simulink model "lab1v3OrozcoBenavides"  (R2017b)
settings: Solver=VariableStepAuto  StartTime=0.0  StopTime=0.01  RelTol=1e-3
undefined symbols (not defined in the file or in its folder): DiscIntNeverNeededParam, magnitude
libraries: commchan3 x8, simulink_extras x7, commrandsrc3 x4, dsparch4 x2, simulink x1, commutil2 x1
settings Model: Creator=n0b0dy  LastModifiedBy=user

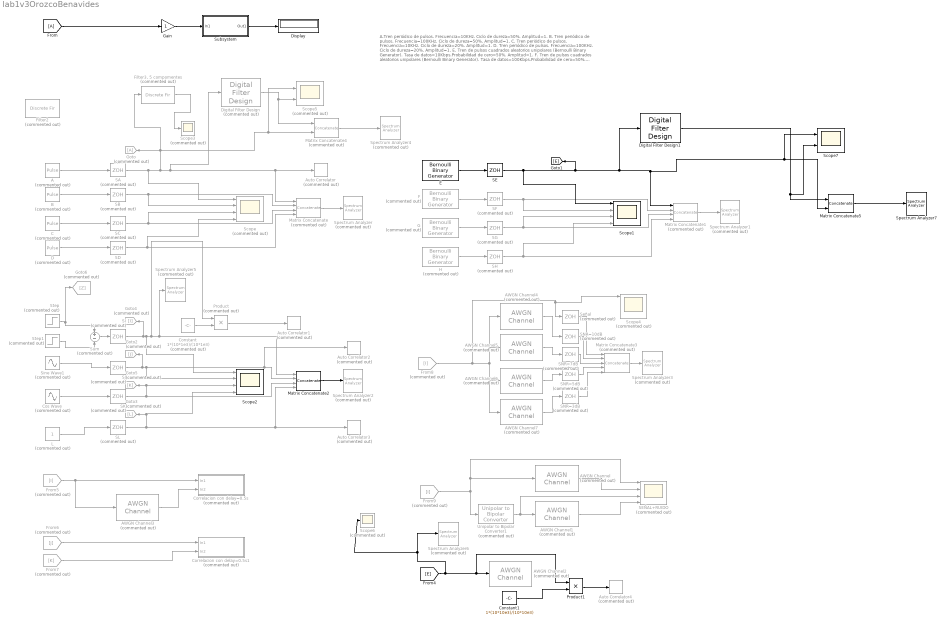
== system lab1v3OrozcoBenavides ==
  note: A.Tren periódico de pulsos. Frecuencia=10KHz. Ciclo de dureza=50%. Amplitud=1.
      | B. Tren periódico de pulsos. Frecuencia=100KHz. Ciclo de dureza=50%. Amplitud=1.
      | C. Tren periódico de pulsos. Frecuencia=10KHz. Ciclo de dureza=20%. Amplitud=1.
      | D. Tren periódico de pulsos. Frecuencia=100KHz. Ciclo de dureza=20%. Amplitud=1.
      | E. Tren de pulsos cuadrados aleatorios unipolares (Bernoulli Binary Generator). Tasa de datos=10Kbps.Probabilidad de cero=50%. Amplitud=1.
      | F. Tren de pulsos cuadrados aleatorios unipolares (Bernoulli Binary Generator). Tasa de datos=100Kbps.Probabilidad de cero=50%. Amplitud=1.
      | G. Tren de pulsos cuadrados aleatorios unipolares (Bernoulli Binary Generator). Tasa de datos=10Kbps.Probabilidad de cero=30%. Amplitud=1.
      | H. Tren de pulsos cuadrados aleatorios unipolares (Bernoulli Binary Generator). Tasa de datos=100Kbps.Probabilidad de cero=30%. Amplitud=1.
      | I. Un pulso rectangular de amplitud 3, iniciando en t0=0.5s y terminando en t1=0.7s
      | J. Seno. Frecuencia=1Khz. Amplitud=1.
      | K. Coseno. Frecuencia=1Khz. Amplitud=1.
      | L. Señal constante. Amplitud=1
  A : DiscretePulseGenerator  Commented=on  PulseType=Time based  Period=1/10E3  PulseWidth=50
  AWGN Channel{,1..2,6} (4 alike) : commchan3/AWGN Channel  Commented=on  InputProcessing=Columns as channels (frame based)  seed=67  noiseMode="Signal to noise ratio  (SNR)"  EbNodB=10  EsNodB=10  SNRdB=10  bitsPerSym=1  Ps=1  Tsym=1  variance=1
  AWGN Channel3 : commchan3/AWGN Channel  Commented=on  InputProcessing=Columns as channels (frame based)  seed=67  noiseMode="Signal to noise ratio  (SNR)"  EbNodB=10  EsNodB=10  SNRdB=5  bitsPerSym=1  Ps=1  Tsym=1  variance=1
  AWGN Channel4 : commchan3/AWGN Channel  Commented=on  InputProcessing=Columns as channels (frame based)  seed=67  noiseMode="Signal to noise ratio  (SNR)"  EbNodB=10  EsNodB=10  SNRdB=30  bitsPerSym=1  Ps=1  Tsym=1  variance=1
  AWGN Channel5 : commchan3/AWGN Channel  Commented=on  InputProcessing=Columns as channels (frame based)  seed=67  noiseMode="Signal to noise ratio  (SNR)"  EbNodB=10  EsNodB=10  SNRdB=20  bitsPerSym=1  Ps=1  Tsym=1  variance=1
  AWGN Channel7 : commchan3/AWGN Channel  Commented=on  InputProcessing=Columns as channels (frame based)  seed=67  noiseMode="Signal to noise ratio  (SNR)"  EbNodB=10  EsNodB=10  SNRdB=3  bitsPerSym=1  Ps=1  Tsym=1  variance=1
  Auto Correlator : simulink_extras/Additional Sinks/Auto Correlator  Commented=on  npts=1000  HowOften=50  sampleT=1/(10*100e3)
      settings: SourceProductName=Simulink  SourceProductBaseCode=SL
  Auto Correlator1 : simulink_extras/Additional Sinks/Auto Correlator  Commented=on  npts=10000  HowOften=100  sampleT=1/(10*1e3)
      settings: SourceProductName=Simulink  SourceProductBaseCode=SL
  Auto Correlator2 : simulink_extras/Additional Sinks/Auto Correlator  Commented=on  npts=1000  HowOften=50  sampleT=1/(10*100e3)
      settings: SourceProductName=Simulink  SourceProductBaseCode=SL
  Auto Correlator3 : simulink_extras/Additional Sinks/Auto Correlator  Commented=on  npts=1000  HowOften=50  sampleT=1/(10*100e3)
      settings: SourceProductName=Simulink  SourceProductBaseCode=SL
  Auto Correlator4 : simulink_extras/Additional Sinks/Auto Correlator  Commented=on  npts=0.01*(1*100e3)  HowOften=50  sampleT=1/(1*1*100e3)
      settings: SourceProductName=Simulink  SourceProductBaseCode=SL
  B : DiscretePulseGenerator  Commented=on  PulseType=Time based  Period=1/100E3  PulseWidth=50  VectorParams1D=off
  C : DiscretePulseGenerator  Commented=on  PulseType=Time based  Period=1/10E3  PulseWidth=20
  Constant : Constant  Commented=on  Value=1*(10*1e3)/(10*1e3)
  Constant1 : Constant  Value=1*(10*10e3)/(10*10e3)  VectorParams1D=off
  Correlacion con delay=0.5s : Subsystem  Commented=on
  Correlacion con delay=0.5s1 : Subsystem  Commented=on
  Cos Wave : Sin  Commented=on  Frequency=1e3*2*pi  Phase=pi/2  SampleTime=0
      settings: AttributesFormatString=|
      | Frecuency = %<Frequency>
      | Phase = %<Phase>
  D : DiscretePulseGenerator  Commented=on  PulseType=Time based  Period=1/100E3  PulseWidth=20
  Digital Filter Design : dsparch4/Digital Filter Design  Commented=on  mwdsp_browser_bugfix_var=off
  Digital Filter Design1 : dsparch4/Digital Filter Design  mwdsp_browser_bugfix_var=off
  Display : Display
  E : commrandsrc3/Bernoulli Binary Generator  ProbabilityOfZero=0.5  SeedSource=Parameter  Seed=1  SampleTime=1/10e3  SamplesPerFrame=1  OutputDataType=double  SimulateUsing=Interpreted execution
  F : commrandsrc3/Bernoulli Binary Generator  Commented=on  ProbabilityOfZero=0.5  SeedSource=Parameter  Seed=1  SampleTime=1/100e3  SamplesPerFrame=1  OutputDataType=double  SimulateUsing=Interpreted execution
  Filter2 : DiscreteFir  Tag=BlockMethodSubSystem  Commented=on  Coefficients=[4.38046656654841762e-05 -4.19168130119133766e-05 -0.000121386266707471151 -0.000265005595843999426 -0.000483929880286931749 -0.000785385479719208899 -0.00116838844519587498 -0.00162088820335549262 -0.00211837965652547384 -0.00262429357472941226 -0.00309240365472468167 -0.00347122798063446373 -0.00371006783715153651 -0.00376598322946659425 -0.00361073126809461058 -0.00323657020863689316 -0.00265988372117567868 -0.00192179242455310867 -0.0010852856491014634 -0.00022892390698464615 0.000562294725985832723 0.00120774054573818891 0.00164212245751450933 0.00182496514804559294 0.00174706032403629556 0.00143270722359442582 0.000937104908236654197 0.000339052776177651075 -0.000270104760592205389 -0.000799685490012579732 -0.00117307419834991686 -0.00133925511256620996 -0.00128052437133370218 -0.00101496544346531812 -0.000593223360786295406 -9.0098624979057212e-05 0.000407829194517540707 0.000816694288465465027 0.00106938093719796613 0.00112654488019772563 0.000983116680090515612 0.000669141685305301489 0.00024377150117316118 -0.000214758300947622162 -0.000623487590944115191 -0.000909288837690687825 -0.00102201616435767173 -0.000943413362638917743 -0.000690311975732371729 -0.000311465081635695193 0.000121453079804872499 0.00052708206831504254 0.000829449660208835633 0.000972112086423019693 0.000928722856611384137 0.000708038562495666934 0.00035238423342301195 -7.02068138446367679e-05 -0.000478776573891657922 -0.000794771976519680653 -0.000957046001095245339 -0.000933662118462325703 -0.000728248932484220615 -0.000379610497823254576 4.54286116717556512e-05 0.000464658782034540541 0.000796232383327042433 0.000974517717138466389 0.000963043704093518205 0.000761969046616292785 0.000408519220074084644 -2.97864715487908991e-05 -0.000467887789648414529 -0.000819563639488438372 -0.00101432965399111214 -0.00101150391553276719 -0.000808641445645382493 -0.000442668221679458384 1.6698949341005064e-05 0.000480169323467016101 0.000856099681400842899 0.00106849485655577544 0.00107239752966509748 0.000863216093056568077 0.000478532571955423607 -8.60809240804113552e-06 -0.000503407751857083523 -0.000907686399168791875 -0.0011392594249544695 -0.00114856463830354406 -0.000929178426529089297 -0.000519999891673953796 1.51181938939170573e-06 0.000533896501371516527 0.00097133288833494509 0.0012245805461409149 0.00123909814434492219 0.0010066725610375592 0.000568096844458311576 6.15874647942870259e-06 -0.000569874227150696309 -0.00104541265328059597 -0.00132325090323160322 -0.00134334704820137252 -0.00109565562907119017 -0.000623315109519916944 -1.53182880747693627e-05 0.000610154722245020639 0.00112861326675984738 0.00143393666346508628 0.00145999600900222916 0.0011948377344181936 0.000684389295089147978 2.46964901632145642e-05 -0.000656013445546513091 -0.00122214672216798808 -0.00155766341892300841 -0.00158973766434169941 -0.00130438657377089369 -0.000750766270524873161 -3.29110235709409793e-05 0.000709675786849656935 0.0013289844717842606 0.00169793347953696959 0.00173626328057938399 0.00142784176525678741 0.000825501436989571993 4.22734076420392036e-05 -0.000769681624686397153 -0.00144850220814824685 -0.00185476672860425212 -0.00189998302907449178 -0.00156563482999592441 -0.000908729359524553838 -5.23786476597378915e-05 0.000837102120019716654 0.00158235004436164386 0.00203017189497679698 0.00208286726094366638 0.00171929023235925407 0.00100113756502400873 6.28249433195016339e-05 -0.000913475729138999142 -0.0017330252814185675 -0.00222720156302766469 -0.00228800099709282074 -0.00189133702366649269 -0.00110418201937342603 -7.36611723914431193e-05 0.00100021303198232826 0.00190316445848833426 0.00244920291234219673 0.00251870603996510057 0.00208427954227722754 0.0012188517116007633 8.39018161508939329e-05 -0.00110038389359039084 -0.00209759709626851235 -0.00270205491143405731 -0.00278093116536051385 -0.00230303831169035265 -0.00134804930342949272 -9.37665819527546183e-05 0.00121662908351330944 0.00232145711129587429 0.00299245975452155271 ...(+8045 chars)]  InputProcessing=Columns as channels (frame based)
  "Filter3, 5 compomentes" : DiscreteFir  Tag=BlockMethodSubSystem  Commented=on  Coefficients=[2.79989185012177059e-05 -0.000105953724690452253 -0.000292454303464867048 -0.000626193909028600372 -0.00112189499276038607 -0.00177137850885229157 -0.00253071916030403942 -0.00331769613747110977 -0.00401905086517821784 -0.00450759844196932467 -0.00466679658214582804 -0.00441810008141596371 -0.00374460911899705384 -0.0027045308751120589 -0.00142938281618603855 -0.000105211597033487704 0.00106091844277730733 0.00188261724507192353 0.0022348413072214527 0.0020835183521437841 0.00149614751761707396 0.000629321570530913597 -0.000305119435651505556 -0.00108814220471705283 -0.00154430269565517366 -0.00158278844786753831 -0.00121802378211626687 -0.000564190059464299482 0.000195607639512460849 0.000857694248338263356 0.0012512554007840411 0.00128263056347404465 0.000958786552950189642 0.000383262236423445373 -0.000274199337726034999 -0.000825960673960223824 -0.00111909902657287121 -0.00107801703422790254 -0.000724561917723311817 -0.000170101675364089743 0.000418017207139567346 0.000865697405373802033 0.0010434894192694593 0.000903814509209919527 0.000494332078311386885 -5.71351389593617321e-05 -0.000581766655390131759 -0.000920498829788223222 -0.000972271144771941426 -0.000724122981004119413 -0.000254944607092817915 0.000289067858801462184 0.000739266533072509128 0.000956536712688483876 0.00087413579753808457 0.000518475369587088376 1.01969522285767357e-06 -0.000516124840445947178 -0.000870633715201949744 -0.000950648066895526779 -0.000730130453763766529 -0.000277523389284990479 0.000265104167651098572 0.000726298236616406811 0.000959050283613696033 0.000887539849975970698 0.00053184298328664214 2.61312754760789659e-06 -0.000533070102660583339 -0.000904109271300230816 -0.000989826233994362372 -0.000759091543592910309 -0.000281516965869250187 0.000293355859759349678 0.00078260479796927161 0.00102793716728616477 0.000946752679220866974 0.000559848451915482192 -1.35289045187603474e-05 -0.000592174508425513386 -0.000990046250571080012 -0.00107589732578213318 -0.00081644516914374291 -0.000288929525607793886 0.000341617329249163367 0.000873847888875211795 0.00113410351522393992 0.00103303002066397584 0.000595957799675754583 -4.28113655282286981e-05 -0.000681112833007499886 -0.00111267784154058815 -0.00119361968305066761 -0.00089021668448018064 -0.000292198959565528296 0.00041351895387779341 0.00100108492215386039 0.00127782046432451703 0.00114724305845931209 0.000642443794521678838 -8.16535047065313006e-05 -0.000795606667856096081 -0.00126796475042223467 -0.0013401100370218405 -0.000979307442644656396 -0.00029227709093609033 0.00050604738013228668 0.00115953993822761996 0.00145283333726422734 0.00128207429085145253 0.000691275250160187471 -0.000138340380323460313 -0.00094369704061957754 -0.00146309449967240313 -0.0015210770939481338 -0.00108743002607618604 -0.000290586108468933338 0.000620045114702857947 0.00135190861876987429 0.00166310951039600071 0.00144210821626320927 0.000747210068665114715 -0.000208038831820198323 -0.00112017805961993518 -0.00169198437246395714 -0.00172905606454615605 -0.00120556060096278176 -0.000276925111661155551 0.000765880737659720341 0.00158728482198131158 0.00191487811821521828 0.00162946894409729472 0.000807808155745899387 -0.000297221137432102773 -0.00133405308442731407 -0.00196402975954140455 -0.00197170100206701037 -0.00133808355744471506 -0.0002520458629370249 0.000945485654472029988 0.0018682142453974363 0.00220875745757978569 0.00184065454238679384 0.000864363128318641999 -0.000419217153904169351 -0.00160107075510280863 -0.00229404430220955021 -0.0022592939518638719 -0.00148803265097405919 -0.000210754428387598407 0.00117104718449970754 0.00221064543398562935 0.00256008141789546831 0.00208611543280144609 0.000919626724432985707 -0.000579437668080587842 -0.00193260400964896336 -0.00269512240175859069 -0.00260163177605153778 -0.00165768833341076388 -0.000145860333272162189 0.00145812159837608256 0.00263448871226449341 0.00298728424072897646 0.00237693078973773807 0.000973325553437070731 ...(+8027 chars)]  InputProcessing=Columns as channels (frame based)
  From5 : From  Commented=on  GotoTag=I
  From6 : From  Commented=on  GotoTag=J
  From7 : From  Commented=on  GotoTag=K
  From8 : From  Commented=on  GotoTag=I
  From9 : From  Commented=on  GotoTag=I
  G : commrandsrc3/Bernoulli Binary Generator  Commented=on  ProbabilityOfZero=0.3  SeedSource=Parameter  Seed=1  SampleTime=1/10e3  SamplesPerFrame=1  OutputDataType=double  SimulateUsing=Interpreted execution
  Gain : Gain
  Goto : Goto  Commented=on
  Goto2 : Goto  Commented=on  GotoTag=J
  Goto3 : Goto  Commented=on  GotoTag=L
  Goto4 : Goto  Commented=on  GotoTag=I
  Goto5 : Goto  Commented=on  GotoTag=K
  Goto6 : Goto  Commented=on  GotoTag=Z
  H : commrandsrc3/Bernoulli Binary Generator  Commented=on  ProbabilityOfZero=0.3  SeedSource=Parameter  Seed=1  SampleTime=1/100e3  SamplesPerFrame=1  OutputDataType=double  SimulateUsing=Interpreted execution
  L : Constant  Commented=on  SampleTime=1/(6*(1000*2*pi))
  Matrix Concatenate : Concatenate  Commented=on  NumInputs=4  Mode=Multidimensional array  ConcatenateDimension=2
  Matrix Concatenate1 : Concatenate  Commented=on  NumInputs=4  Mode=Multidimensional array  ConcatenateDimension=2
  Matrix Concatenate2 : Concatenate  NumInputs=4  Mode=Multidimensional array  ConcatenateDimension=2
  Matrix Concatenate3 : Concatenate  Commented=on  NumInputs=5  Mode=Multidimensional array  ConcatenateDimension=2
  Matrix Concatenate4 : Concatenate  Commented=on  Mode=Multidimensional array  ConcatenateDimension=2
  Matrix Concatenate5 : Concatenate  Mode=Multidimensional array  ConcatenateDimension=2
  Product : Product  Commented=on
  Product1 : Product
  SA : ZeroOrderHold  Commented=on  SampleTime=1/(10*100e3)
  SB : ZeroOrderHold  Commented=on  SampleTime=1/(10*100e3)
  SC : ZeroOrderHold  Commented=on  SampleTime=1/(10*100e3)
  SD : ZeroOrderHold  Commented=on  SampleTime=1/(10*100e3)
  SE : ZeroOrderHold  SampleTime=1/(10e3*100)
  SEÑAL+RUIDO : Scope  Commented=on  NumInputPorts=4
  SF : ZeroOrderHold  Commented=on  SampleTime=1/(10*100e3)
  SG : ZeroOrderHold  Commented=on  SampleTime=1/(10*100e3)
  SH : ZeroOrderHold  Commented=on  SampleTime=1/(10*100e3)
  SI : ZeroOrderHold  Commented=on  SampleTime=1/(1e3)
  SJ : ZeroOrderHold  Commented=on  SampleTime=1/(1*100e3)
  SK : ZeroOrderHold  Commented=on  SampleTime=1/(10*100e3)
  SL : ZeroOrderHold  Commented=on  SampleTime=1/(1*100e3)
  SNR=10dB : ZeroOrderHold  Commented=on  SampleTime=1/(1*1e3)
  SNR=3dB : ZeroOrderHold  Commented=on  SampleTime=1/(1*1e3)
  SNR=5dB : ZeroOrderHold  Commented=on  SampleTime=1/(1*1e3)
  SNR=7dB : ZeroOrderHold  Commented=on  SampleTime=1/(1*1e3)
  Scope : Scope  Commented=on  NumInputPorts=4
  Scope1 : Scope  NumInputPorts=4
  Scope2 : Scope  NumInputPorts=4
  Scope3 : Scope  Commented=on
  Scope4 : Scope  Commented=on  NumInputPorts=4
  Scope5 : Scope  Commented=on  NumInputPorts=2
  Scope6 : Scope  Commented=on
  Scope7 : Scope  NumInputPorts=2
  Señal : ZeroOrderHold  Commented=on  SampleTime=1/(1*1e3)
  Sine Wave1 : Sin  Commented=on  Frequency=1e3*2*pi  SampleTime=0
      settings: AttributesFormatString=|
      | Frecuency = %<Frequency>
      | Phase = %<Phase>
  Spectrum Analyzer{,1..6} (7 alike) : SpectrumAnalyzer  Commented=on
  Spectrum Analyzer7 : SpectrumAnalyzer
  Step : Step  Commented=on  Time=0.5  After=3  SampleTime=1e-3
      settings: AttributesFormatString=Step Time = %<Time>
  Step1 : Step  Commented=on  Time=0.7  After=3  SampleTime=1e-3
      settings: AttributesFormatString=Step Time = %<Time>
  Subsystem : Subsystem
  Sum : Sum  Commented=on  Inputs=+|-
  Unipolar to Bipolar Converter1 : commutil2/Unipolar to Bipolar Converter  Commented=on  M=2  polarity=Positive  dataType=Inherit via internal rule
      settings: SourceProductName=Communications System Toolbox
  wires:
  A/1 -> SA/1
  E/1 -> SE/1
  F/1 -> SF/1
  G/1 -> SG/1
  H/1 -> SH/1
  B/1 -> SB/1
  C/1 -> SC/1
  D/1 -> SD/1
  SA/1 -> Scope/1, Scope5/1, Matrix Concatenate4/2, "Filter3, 5 compomentes"/1, Goto/1, Digital Filter Design/1, Auto Correlator/1, Matrix Concatenate/1
  SD/1 -> Matrix Concatenate/4, Scope/4
  SH/1 -> Matrix Concatenate1/4, Scope1/4
  SG/1 -> Matrix Concatenate1/3, Scope1/3
  SF/1 -> Matrix Concatenate1/2, Scope1/2
  Matrix Concatenate1/1 -> Spectrum Analyzer1/1
  SC/1 -> Scope/3, Matrix Concatenate/3
  SB/1 -> Scope/2, Matrix Concatenate/2
  L/1 -> SL/1
  Sine Wave1/1 -> SJ/1
  Cos Wave/1 -> SK/1
  SI/1 -> Goto4/1, Scope2/1, Product/1, Spectrum Analyzer5/1, Matrix Concatenate2/1
  SJ/1 -> Goto2/1, Scope2/2, Auto Correlator2/1, Matrix Concatenate2/2
  SK/1 -> Goto5/1, Scope2/3, Matrix Concatenate2/3
  SL/1 -> Goto3/1, Scope2/4, Auto Correlator3/1, Matrix Concatenate2/4
  Matrix Concatenate2/1 -> Spectrum Analyzer2/1
  Matrix Concatenate/1 -> Spectrum Analyzer/1
  [A] -> Gain/1
  Gain/1 -> Subsystem/1(In1)
  Subsystem/1(Out1) -> Display/1
  AWGN Channel/1 -> SEÑAL+RUIDO/2
  Unipolar to Bipolar Converter1/1 -> SEÑAL+RUIDO/3, AWGN Channel1/1
  AWGN Channel1/1 -> SEÑAL+RUIDO/4
  Step1/1 -> Sum/2
  Step/1 -> Goto6/1, Sum/1
  Sum/1 -> SI/1
  Constant/1 -> Product/2
  Product/1 -> Auto Correlator1/1
  Constant1/1 -> Product1/2
  Product1/1 -> Auto Correlator4/1
  [E] -> Scope6/1, Spectrum Analyzer6/1, Product1/1, AWGN Channel2/1
  From5/1 -> AWGN Channel3/1, Correlacion con delay=0.5s/1(In1)
  AWGN Channel3/1 -> Correlacion con delay=0.5s/2(In2)
  From6/1 -> Correlacion con delay=0.5s1/1(In1)
  From7/1 -> Correlacion con delay=0.5s1/2(In2)
  Matrix Concatenate3/1 -> Spectrum Analyzer3/1
  From8/1 -> AWGN Channel4/1, AWGN Channel5/1, AWGN Channel6/1, AWGN Channel7/1, Scope4/1, Señal/1
  AWGN Channel4/1 -> SNR=10dB/1
  AWGN Channel5/1 -> SNR=7dB/1
  AWGN Channel6/1 -> SNR=5dB/1
  AWGN Channel7/1 -> SNR=3dB/1
  Señal/1 -> Matrix Concatenate3/1
  SNR=10dB/1 -> Matrix Concatenate3/2
  SNR=7dB/1 -> Matrix Concatenate3/3
  SNR=5dB/1 -> Matrix Concatenate3/4
  SNR=3dB/1 -> Matrix Concatenate3/5
  From9/1 -> Unipolar to Bipolar Converter1/1, AWGN Channel/1, SEÑAL+RUIDO/1
  "Filter3, 5 compomentes"/1 -> Scope3/1
  Matrix Concatenate4/1 -> Spectrum Analyzer4/1
  Digital Filter Design/1 -> Scope5/2, Matrix Concatenate4/1
  Digital Filter Design1/1 -> Scope7/2, Matrix Concatenate5/1
  Matrix Concatenate5/1 -> Spectrum Analyzer7/1
  SE/1 -> [E], Digital Filter Design1/1, Matrix Concatenate5/2, Scope7/1, Matrix Concatenate1/1, Scope1/1

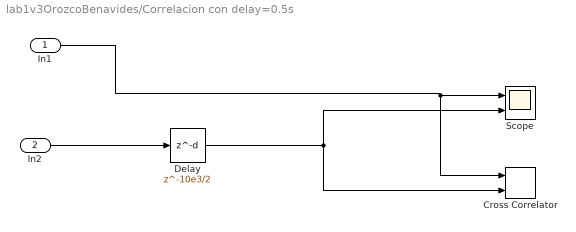
== system lab1v3OrozcoBenavides/Correlacion con delay=0.5s ==
  In1 : Inport
  In2 : Inport  Port=2
  Cross Correlator : simulink_extras/Additional Sinks/Cross Correlator  npts=2*(10*1e3)  HowOften=50  sampleT=1/(10*1e3)
      settings: SourceProductName=Simulink  SourceProductBaseCode=SL
  Delay : Delay  DelayLength=10e3/2  InitialCondition=0
  Scope : Scope  NumInputPorts=2
  wires:
  In1/1 -> Cross Correlator/1, Scope/1
  Delay/1 -> Cross Correlator/2, Scope/2
  In2/1 -> Delay/1

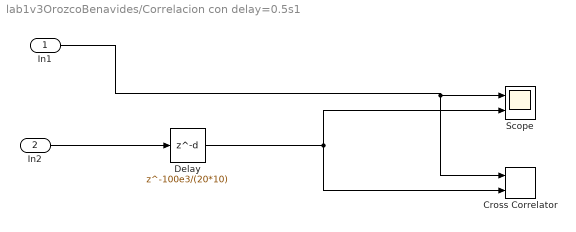
== system lab1v3OrozcoBenavides/Correlacion con delay=0.5s1 ==
  In1 : Inport
  In2 : Inport  Port=2
  Cross Correlator : simulink_extras/Additional Sinks/Cross Correlator  npts=0.01*(1*100e3)  HowOften=50  sampleT=1/(100*1e3)
      settings: SourceProductName=Simulink  SourceProductBaseCode=SL
  Delay : Delay  DelayLength=100e3/(20*10)  InitialCondition=0
  Scope : Scope  NumInputPorts=2
  wires:
  In1/1 -> Cross Correlator/1, Scope/1
  Delay/1 -> Cross Correlator/2, Scope/2
  In2/1 -> Delay/1

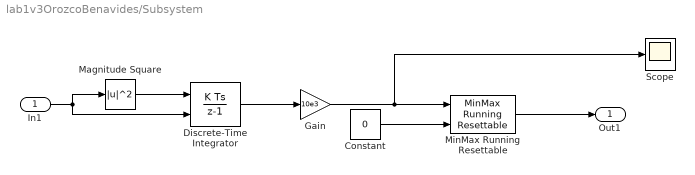
== system lab1v3OrozcoBenavides/Subsystem ==
  In1 : Inport
  Constant : Constant  Value=0
  Discrete-Time Integrator : DiscreteIntegrator  gainval=1  ExternalReset=rising  InitialConditionSetting=State (most efficient)  SampleTime=-1  ICPrevOutput=DiscIntNeverNeededParam  ICPrevScaledInput=DiscIntNeverNeededParam
  Gain : Gain  Gain=10e3
  Magnitude Square : Math  Operator=magnitude^2  RndMeth=Zero  SaturateOnIntegerOverflow=on
  MinMax Running Resettable : simulink/Math Operations/MinMax Running Resettable  Function=max  vinit=0.0
  Scope : Scope
  Out1 : Outport
  wires:
  In1/1 -> Discrete-Time Integrator/2, Magnitude Square/1
  MinMax Running Resettable/1 -> Out1/1
  Gain/1 -> Scope/1, MinMax Running Resettable/1
  Constant/1 -> MinMax Running Resettable/2
  Magnitude Square/1 -> Discrete-Time Integrator/1
  Discrete-Time Integrator/1 -> Gain/1
